simulink model "VFOC"  (R2015a)
settings: Solver=ode45  StartTime=0.0  StopTime=10.0  RelTol=1e-3
values from neighbouring files (symbols this model uses):
  C = 2350e-6    (= 0.00235)    [VOC_param.m]    (also in VOC_param_paper.m = 0.0022; controller_parameters.m = 0.0022; power_control_param.m = 0.02)
  Hp = 0    [VOC_param.m]    (also in power_control_param.m = 20)
  Hq = 0    [VOC_param.m]    (also in power_control_param.m)
  I = 0.1    [power_control_param.m]
  Ka = fluxeff    (= 0.15)    [VOC_param.m]    (also in VOC_param_paper.m; power_control_param.m)
  L = 8e-3    (= 0.008)    [VOC_param.m]    (also in VOC_param_paper.m = 0.003; controller_parameters.m = 0.003; current_controller_param.m = 0.005; power_control_param.m = 0.1)
  p = 4    [VOC_param.m]    (also in VOC_param_paper.m; power_control_param.m)
  P = 1    [power_control_param.m]
  R = 0.1    [VOC_param.m]    (also in VOC_param_paper.m = 0.05; controller_parameters.m = 0.05; current_controller_param.m; power_control_param.m = 0)
  RL = 120    [VOC_param.m]    (also in VOC_param_paper.m = 150; power_control_param.m = 80)
  rpm2radps = pi/30    (= 0.10471975512)    [VOC_param.m]    (also in VOC_param_paper.m; power_control_param.m)
  U = 311    [VOC_param.m]    (also in power_control_param.m)
  Udcref = 120    [VOC_param.m]    (also in VOC_param_paper.m; power_control_param.m = 10)
  w = 2*pi*f    (= 314.159265359)    [VOC_param.m]    (also in controller_parameters.m; current_controller_param.m; power_control_param.m)
libraries: simulink x2
settings Model: Creator=rblan  LastModifiedBy=rblan

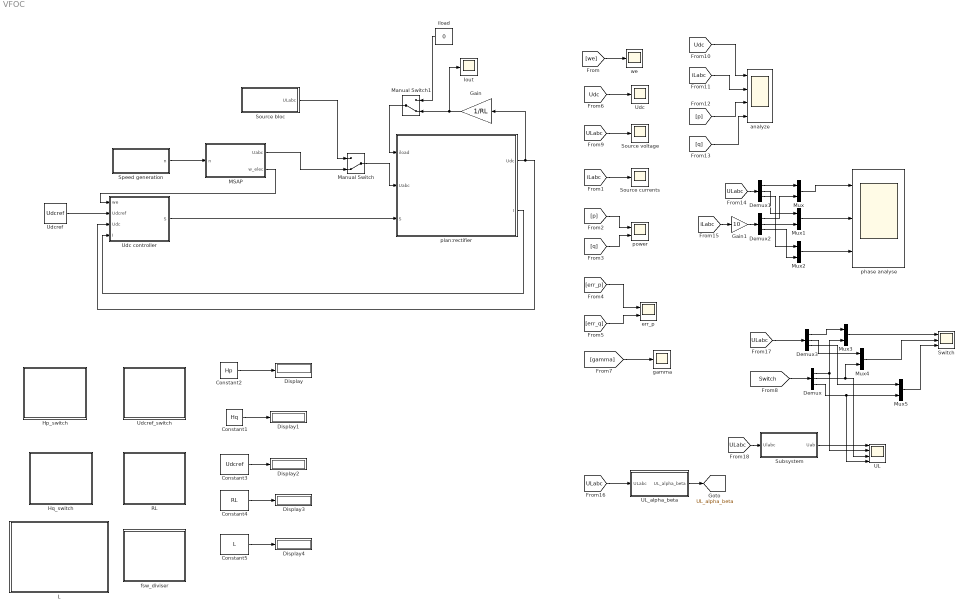
== system VFOC ==
  Constant1 : Constant  Value=Hq
  Constant2 : Constant  Value=Hp
  Constant3 : Constant  Value=Udcref
  Constant4 : Constant  Value=RL
  Constant5 : Constant  Value=L
  Demux{,1..3} (4 alike) : Demux  Outputs=3
  Display{,1..4} (5 alike) : Display
  Gain : Gain  Gain=1/RL
  Gain1 : Gain  Gain=10
  Hp_switch : Subsystem  DialogController=hmiCreateDDGDialog  IsWebBlock=on  mask(MathWorksWebBlock){webBlockId=fe3dbe73-a954-44d9-9dcb-6f2e0f6423d3, webBlockType=continuousknob, ShowInLibBrowser=on, ShowInitialText=on, HMISrcModelName=VFOC}
      mask prompts: webBlockId "WebBlock Id"; webBlockType "WebBlock Type"; HMISrcModelName "Source Model"
      mask Help: helpview([docroot '/mapfiles/simulink.map'], 'hmi_knob')
      mask Display:
      | if strcmp(get_param(bdroot(gcb),'BlockDiagramType'), 'library')
      |     image([(matlabroot) '/toolbox/simulink/hmi/icons/ContinuousKnob.png']);
      | end
  Hq_switch : Subsystem  DialogController=hmiCreateDDGDialog  IsWebBlock=on  mask(MathWorksWebBlock){webBlockId=a89797ed-0246-4893-8a6d-d9668782cbd3, webBlockType=continuousknob, ShowInLibBrowser=on, ShowInitialText=on, HMISrcModelName=VFOC}
      mask prompts: webBlockId "WebBlock Id"; webBlockType "WebBlock Type"; HMISrcModelName "Source Model"
      mask Help: helpview([docroot '/mapfiles/simulink.map'], 'hmi_knob')
      mask Display:
      | if strcmp(get_param(bdroot(gcb),'BlockDiagramType'), 'library')
      |     image([(matlabroot) '/toolbox/simulink/hmi/icons/ContinuousKnob.png']);
      | end
  Iout : Scope
      settings: YMin=0.2275  YMax=0.2575  SaveName=ScopeData13
  L : Subsystem  DialogController=hmiCreateDDGDialog  IsWebBlock=on  mask(MathWorksWebBlock){webBlockId=ffd7f022-e8a1-4d04-9927-9b962ba217d4, webBlockType=continuousknob, ShowInLibBrowser=on, ShowInitialText=on, HMISrcModelName=VFOC}
      mask prompts: webBlockId "WebBlock Id"; webBlockType "WebBlock Type"; HMISrcModelName "Source Model"
      mask Help: helpview([docroot '/mapfiles/simulink.map'], 'hmi_knob')
      mask Display:
      | if strcmp(get_param(bdroot(gcb),'BlockDiagramType'), 'library')
      |     image([(matlabroot) '/toolbox/simulink/hmi/icons/ContinuousKnob.png']);
      | end
  MSAP : Subsystem
  Manual Switch : ManualSwitch  CurrentSetting=0
  Manual Switch1 : ManualSwitch  CurrentSetting=0
  Mux{,1..5} (6 alike) : Mux  Inputs=2
  RL : Subsystem  DialogController=hmiCreateDDGDialog  IsWebBlock=on  mask(MathWorksWebBlock){webBlockId=6d3a3d3f-09f6-4f12-a865-f4fdcd28252a, webBlockType=continuousknob, ShowInLibBrowser=on, ShowInitialText=on, HMISrcModelName=VFOC}
      mask prompts: webBlockId "WebBlock Id"; webBlockType "WebBlock Type"; HMISrcModelName "Source Model"
      mask Help: helpview([docroot '/mapfiles/simulink.map'], 'hmi_knob')
      mask Display:
      | if strcmp(get_param(bdroot(gcb),'BlockDiagramType'), 'library')
      |     image([(matlabroot) '/toolbox/simulink/hmi/icons/ContinuousKnob.png']);
      | end
  Source bloc : Subsystem
  Source currents : Scope
      settings: TimeRange=2  YMin=-3  YMax=2.25  SaveName=Iabc
  "Source voltage " : Scope
      settings: TimeRange=0.06239913932221623  YMin=-20  YMax=20  SaveName=Uabc
  Speed generation : Subsystem
  Subsystem : Subsystem
  Switch : Scope  NumInputPorts=3
      settings: YMin=-2~-5~-5  YMax=5~5~5  SaveName=ScopeData8
  "UL " : Scope  NumInputPorts=4
      settings: YMin=-2~-5~-5~-5  YMax=5~5~5~5  SaveName=ScopeData19
  UL_alpha_beta : Subsystem
  Udc : Scope
      settings: TimeRange=3  YMin=15  YMax=21.5  SaveName=Udc
  Udc controller : Subsystem
  Udcref : Constant  Value=Udcref
  Udcref_switch : Subsystem  DialogController=hmiCreateDDGDialog  IsWebBlock=on  mask(MathWorksWebBlock){webBlockId=8174ab9b-ad42-417a-b04d-5b98e4451fc4, webBlockType=continuousknob, ShowInLibBrowser=on, ShowInitialText=on, HMISrcModelName=VFOC}
      mask prompts: webBlockId "WebBlock Id"; webBlockType "WebBlock Type"; HMISrcModelName "Source Model"
      mask Help: helpview([docroot '/mapfiles/simulink.map'], 'hmi_knob')
      mask Display:
      | if strcmp(get_param(bdroot(gcb),'BlockDiagramType'), 'library')
      |     image([(matlabroot) '/toolbox/simulink/hmi/icons/ContinuousKnob.png']);
      | end
  analyze : Scope  NumInputPorts=4
      settings: TimeRange=0.06239913932221623  YMin=0~-1.75~-25~-5  YMax=20~1.75~100~100  SaveName=Uabc1
  err_p : Scope  NumInputPorts=2
      settings: TimeRange=2  YMin=-40~-65  YMax=40~0  SaveName=err_p
  fsw_diviser : Subsystem  DialogController=hmiCreateDDGDialog  IsWebBlock=on  mask(MathWorksWebBlock){webBlockId=92bd8738-3137-464c-9b2e-3fda7a42618d, webBlockType=continuousknob, ShowInLibBrowser=on, ShowInitialText=on, HMISrcModelName=VFOC}
      mask prompts: webBlockId "WebBlock Id"; webBlockType "WebBlock Type"; HMISrcModelName "Source Model"
      mask Help: helpview([docroot '/mapfiles/simulink.map'], 'hmi_knob')
      mask Display:
      | if strcmp(get_param(bdroot(gcb),'BlockDiagramType'), 'library')
      |     image([(matlabroot) '/toolbox/simulink/hmi/icons/ContinuousKnob.png']);
      | end
  gamma : Scope
      settings: YMin=-2  SaveName=ScopeData5
  iload : Constant  Value=0
  phase analyse : Scope  NumInputPorts=3
      settings: TimeRange=0.06239913932221623  YMin=-30~-30~-30  YMax=30~30~30  SaveName=Uabc2
  plan:rectifier : Subsystem
  "power " : Scope  NumInputPorts=2
      settings: YMin=-20~-5  YMax=75~47.5  SaveName=p
  we : Scope
      settings: YMin=119.381  YMax=131.947  SaveName=ScopeData10
  tag scope: UL_alpha_beta=global
  wires:
  [iLabc] -> Source currents/1
  [p] -> "power "/1
  [q] -> "power "/2
  [err_p] -> err_p/1
  [Udc] -> Udc/1
  [gamma] -> gamma/1
  Manual Switch/1 -> plan:rectifier/2(Uabc)
  [ULabc] -> "Source voltage "/1
  Source bloc/1(ULabc) -> Manual Switch/1
  [we] -> we/1
  Udcref/1 -> Udc controller/2(Udcref)
  plan:rectifier/1(Udc) -> Gain/1, Udc controller/3(Udc)
  MSAP/1(Uabc) -> Manual Switch/2
  Speed generation/1(n) -> MSAP/1(n)
  MSAP/2(w_elec) -> Udc controller/1(we)
  [Switch] -> Demux/1
  plan:rectifier/2(I) -> Udc controller/4(I)
  Udc controller/1(S) -> plan:rectifier/3(S)
  iload/1 -> Manual Switch1/1
  Gain/1 -> Iout/1, Manual Switch1/2
  Manual Switch1/1 -> plan:rectifier/1(iload)
  [Udc] -> analyze/1
  [iLabc] -> analyze/2
  [p] -> analyze/3
  [q] -> analyze/4
  [ULabc] -> Demux1/1
  [iLabc] -> Gain1/1
  Mux/1 -> phase analyse/1
  Demux1/1 -> Mux/1
  Demux2/1 -> Mux/2
  Mux1/1 -> phase analyse/2
  Mux2/1 -> phase analyse/3
  Demux1/2 -> Mux1/1
  Demux2/2 -> Mux1/2
  Demux1/3 -> Mux2/1
  Demux2/3 -> Mux2/2
  Gain1/1 -> Demux2/1
  [err_q] -> err_p/2
  Constant2/1 -> Display/1
  Constant1/1 -> Display1/1
  Constant3/1 -> Display2/1
  Constant4/1 -> Display3/1
  Constant5/1 -> Display4/1
  [ULabc] -> UL_alpha_beta/1(ULabc)
  UL_alpha_beta/1(UL_alpha_beta) -> [UL_alpha_beta]
  [ULabc] -> Demux3/1
  Mux3/1 -> Switch/1
  Demux3/1 -> Mux3/1
  Demux/1 -> Mux3/2, "UL "/2
  Mux4/1 -> Switch/2
  Demux3/2 -> Mux4/1
  Demux/2 -> "UL "/3, Mux4/2
  Mux5/1 -> Switch/3
  Demux3/3 -> Mux5/1
  Demux/3 -> "UL "/4, Mux5/2
  [ULabc] -> Subsystem/1(Ulabc)
  Subsystem/1("Uab ") -> "UL "/1

== system VFOC/Hp_switch ==

== system VFOC/Hq_switch ==

== system VFOC/L ==

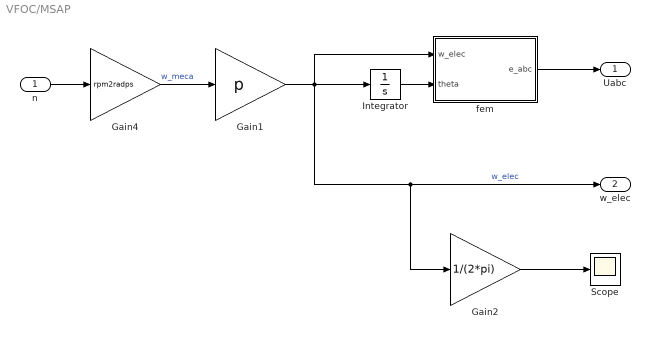
== system VFOC/MSAP ==
  n : Inport
  Gain1 : Gain  Gain=p
  Gain2 : Gain  Gain=1/(2*pi)
  Gain4 : Gain  Gain=rpm2radps
  Integrator : Integrator
  Scope : Scope
      settings: YMin=19  YMax=21  SaveName=ScopeData9
  fem : Subsystem
  Uabc : Outport
  w_elec : Outport  Port=2
  wires:
  Integrator/1 -> fem/2(theta)
  Gain1/1 -> Integrator/1, Gain2/1, w_elec/1, fem/1(w_elec)  "w_elec"
  n/1 -> Gain4/1
  Gain4/1 -> Gain1/1  "w_meca"
  fem/1(e_abc) -> Uabc/1
  Gain2/1 -> Scope/1

== system VFOC/RL ==

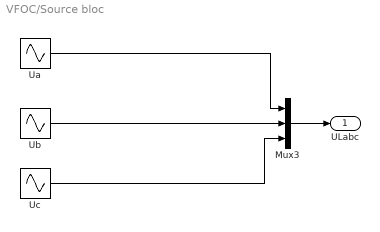
== system VFOC/Source bloc ==
  Mux3 : Mux  Inputs=3
  Ua : Sin  Amplitude=U  Frequency=w  SampleTime=0
  Ub : Sin  Amplitude=U  Frequency=w  Phase=-2*pi/3  SampleTime=0
  Uc : Sin  Amplitude=U  Frequency=w  Phase=-4*pi/3  SampleTime=0
  ULabc : Outport
  wires:
  Ua/1 -> Mux3/1
  Uc/1 -> Mux3/3
  Ub/1 -> Mux3/2
  Mux3/1 -> ULabc/1

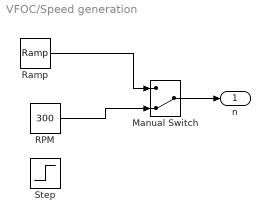
== system VFOC/Speed generation ==
  Manual Switch : ManualSwitch  CurrentSetting=0
  RPM : Constant  Value=300
  Ramp : simulink/Sources/Ramp  slope=50  start=0  X0=100
  Step : Step  Time=1.5  After=0  SampleTime=0
  n : Outport
  wires:
  Ramp/1 -> Manual Switch/1
  Manual Switch/1 -> n/1
  RPM/1 -> Manual Switch/2

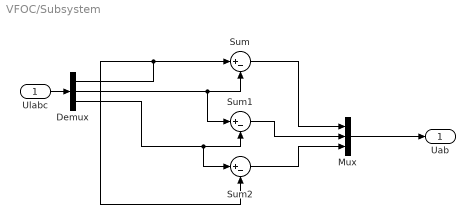
== system VFOC/Subsystem ==
  Ulabc : Inport
  Demux : Demux  Outputs=3
  Mux : Mux  Inputs=3
  Sum : Sum  Inputs=|+-
  Sum1 : Sum  Inputs=|+-
  Sum2 : Sum  Inputs=|+-
  "Uab " : Outport
  wires:
  Ulabc/1 -> Demux/1
  Demux/1 -> Sum/1, Sum2/2
  Demux/2 -> Sum1/1, Sum/2
  Demux/3 -> Sum2/1, Sum1/2
  Mux/1 -> "Uab "/1
  Sum/1 -> Mux/1
  Sum1/1 -> Mux/2
  Sum2/1 -> Mux/3

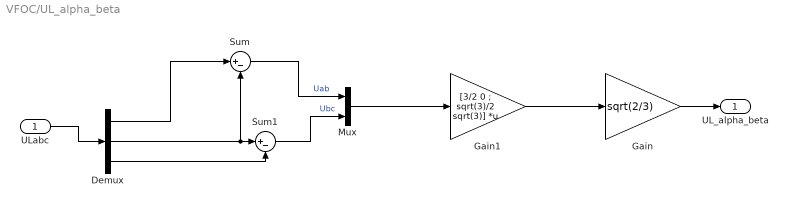
== system VFOC/UL_alpha_beta ==
  ULabc : Inport
  Demux : Demux  Outputs=3
  Gain : Gain  Gain=sqrt(2/3)
  Gain1 : Gain  Gain=[3/2 0 ; sqrt(3)/2 sqrt(3)]  Multiplication=Matrix(K*u)
  Mux : Mux  Inputs=2
  Sum : Sum  Inputs=|+-
  Sum1 : Sum  Inputs=|+-
  UL_alpha_beta : Outport
  wires:
  ULabc/1 -> Demux/1
  Demux/1 -> Sum/1
  Demux/2 -> Sum/2, Sum1/1
  Demux/3 -> Sum1/2
  Gain/1 -> UL_alpha_beta/1
  Gain1/1 -> Gain/1
  Sum/1 -> Mux/1  "Uab"
  Sum1/1 -> Mux/2  "Ubc"
  Mux/1 -> Gain1/1

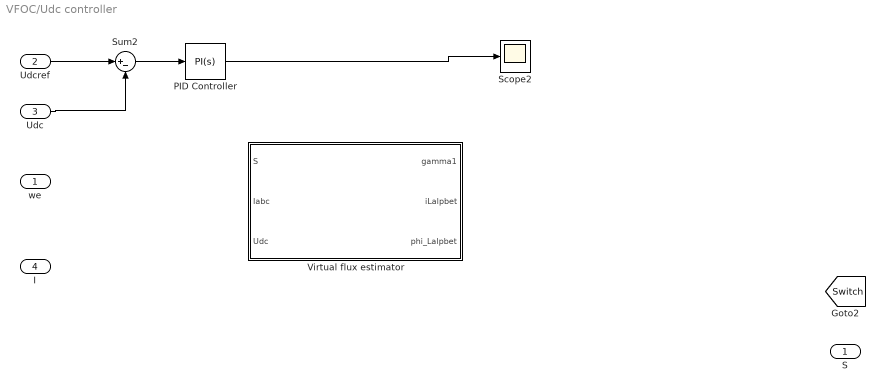
== system VFOC/Udc controller ==
  we : Inport
  Udcref : Inport  Port=2
  Udc : Inport  Port=3
  I : Inport  Port=4
  PID Controller : simulink/Continuous/PID Controller  Controller=PI  TimeDomain=Continuous-time  SampleTime=-1  IntegratorMethod=Forward Euler  FilterMethod=Forward Euler  Form=Parallel  UseFilter=on  ControllerParametersSource=internal  P=P  I=I  D=0  N=100  InitialConditionSource=internal  InitialConditionForIntegrator=0  InitialConditionForFilter=0  ExternalReset=none  LimitOutput=off  UpperSaturationLimit=inf  LowerSaturationLimit=-inf  LinearizeAsGain=on  AntiWindupMode=none  Kb=1  TrackingMode=off  Kt=1  PParamMin=[]  PParamMax=[]  IParamMin=[]  IParamMax=[]  DParamMin=[]  DParamMax=[]  NParamMin=[]  NParamMax=[]  KbParamMin=[]  KbParamMax=[]  KtParamMin=[]  KtParamMax=[]  POutMin=[]  POutMax=[]  IOutMin=[]  IOutMax=[]  DOutMin=[]  DOutMax=[]  NOutMin=[]  NOutMax=[]  KbOutMin=[]  KbOutMax=[]  KtOutMin=[]  KtOutMax=[]  IntegratorOutMin=[]  IntegratorOutMax=[]  FilterOutMin=[]  FilterOutMax=[]  SumOutMin=[]  SumOutMax=[]  SumI1OutMin=[]  SumI1OutMax=[]  SumI2OutMin=[]  SumI2OutMax=[]  SumI3OutMin=[]  SumI3OutMax=[]  SumDOutMin=[]  SumDOutMax=[]  SaturationOutMin=[]  SaturationOutMax=[]  IntegratorContinuousStateAttributes=''  IntegratorStateMustResolveToSignalObject=off  IntegratorRTWStateStorageClass=Auto  FilterContinuousStateAttributes=''  FilterStateMustResolveToSignalObject=off  FilterRTWStateStorageClass=Auto  DifferentiatorICPrevScaledInput=0  DifferentiatorOutMin=[]  DifferentiatorOutMax=[]
  Scope2 : Scope
      settings: YMin=230  YMax=265  SaveName=ScopeData17
  Sum2 : Sum  Inputs=|+-
  Virtual flux estimator : Subsystem
  S : Outport
  tag scope: Switch=global
  wires:
  ? -> S/1, [Switch]
  Udc/1 -> Sum2/2
  Sum2/1 -> PID Controller/1
  Udcref/1 -> Sum2/1
  PID Controller/1 -> Scope2/1

== system VFOC/Udcref_switch ==

== system VFOC/fsw_diviser ==

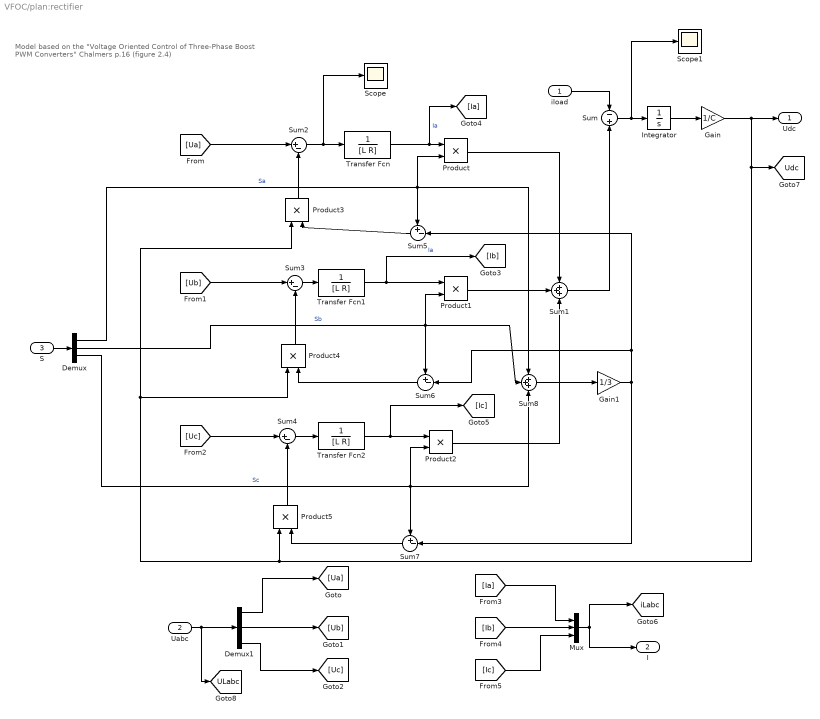
== system VFOC/plan:rectifier ==
  note: Model based on the "Voltage Oriented Control of Three‐Phase
      | Boost PWM Converters" Chalmers p.16 (figure 2.4)
  iload : Inport
  Uabc : Inport  Port=2
  S : Inport  Port=3
  Demux : Demux  Outputs=3
  Demux1 : Demux  Outputs=3
  Gain : Gain  Gain=1/C
  Gain1 : Gain  Gain=1/3
  Integrator : Integrator
  Mux : Mux  Inputs=3
  Product{,1..5} (6 alike) : Product
  Scope : Scope
      settings: SaveName=ScopeData14
  Scope1 : Scope
      settings: SaveName=ScopeData12
  Sum : Sum  Inputs=-|+
  Sum1 : Sum  Inputs=+++
  Sum2 : Sum  Inputs=|+-
  Sum3 : Sum  Inputs=|+-
  Sum4 : Sum  Inputs=|+-
  Sum5 : Sum  Inputs=+-|
  Sum6 : Sum  Inputs=+-|
  Sum7 : Sum  Inputs=+-|
  Sum8 : Sum  Inputs=+++
  Transfer Fcn : TransferFcn  Denominator=[L R]  ContinuousStateAttributes='Ia'
  Transfer Fcn1 : TransferFcn  Denominator=[L R]
  Transfer Fcn2 : TransferFcn  Denominator=[L R]
  Udc : Outport
  I : Outport  Port=2
  tag scope: ULabc=global, Udc=global, iLabc=global
  wires:
  Gain/1 -> [Udc], Product5/1, Product3/1, Product4/1, Udc/1
  Integrator/1 -> Gain/1
  iload/1 -> Sum/1
  Sum1/1 -> Sum/2
  Product/1 -> Sum1/1
  Product1/1 -> Sum1/2
  Product2/1 -> Sum1/3
  Transfer Fcn/1 -> [Ia], Product/1  "Ia"
  Transfer Fcn1/1 -> [Ib], Product1/1  "Ia"
  Transfer Fcn2/1 -> [Ic], Product2/1
  Sum2/1 -> Scope/1, Transfer Fcn/1
  [Ua] -> Sum2/1
  Product3/1 -> Sum2/2
  Sum3/1 -> Transfer Fcn1/1
  Sum4/1 -> Transfer Fcn2/1
  [Ub] -> Sum3/1
  [Uc] -> Sum4/1
  Demux/1 -> Sum8/1, Product/2, Sum5/1  "Sa"
  Demux/2 -> Sum6/1, Sum8/2, Product1/2  "Sb"
  Demux/3 -> Sum8/3, Sum7/1, Product2/2  "Sc"
  Product4/1 -> Sum3/2
  Product5/1 -> Sum4/2
  Sum5/1 -> Product3/2
  Sum6/1 -> Product4/2
  Sum7/1 -> Product5/2
  Sum/1 -> Scope1/1, Integrator/1
  Sum8/1 -> Gain1/1
  Gain1/1 -> Sum6/2, Sum5/2, Sum7/2
  S/1 -> Demux/1
  Uabc/1 -> [ULabc], Demux1/1
  Demux1/1 -> [Ua]
  Demux1/2 -> [Ub]
  Demux1/3 -> [Uc]
  Mux/1 -> [iLabc], I/1
  [Ia] -> Mux/1
  [Ib] -> Mux/2
  [Ic] -> Mux/3

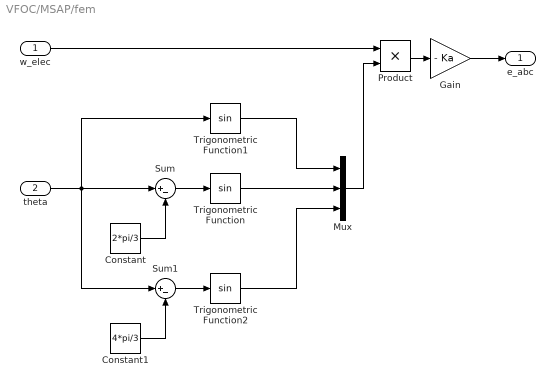
== system VFOC/MSAP/fem ==
  w_elec : Inport
  theta : Inport  Port=2
  Constant : Constant  Value=2*pi/3
  Constant1 : Constant  Value=4*pi/3
  Gain : Gain  Gain=- Ka
  Mux : Mux  Inputs=3
  Product : Product
  Sum : Sum  Inputs=|+-
  Sum1 : Sum  Inputs=|+-
  Trigonometric Function : Trigonometry
  Trigonometric Function1 : Trigonometry
  Trigonometric Function2 : Trigonometry
  e_abc : Outport
  wires:
  Mux/1 -> Product/2
  theta/1 -> Sum/1, Trigonometric Function1/1, Sum1/1
  Constant1/1 -> Sum1/2
  Sum1/1 -> Trigonometric Function2/1
  Constant/1 -> Sum/2
  Sum/1 -> Trigonometric Function/1
  w_elec/1 -> Product/1
  Product/1 -> Gain/1
  Gain/1 -> e_abc/1
  Trigonometric Function1/1 -> Mux/1
  Trigonometric Function2/1 -> Mux/3
  Trigonometric Function/1 -> Mux/2

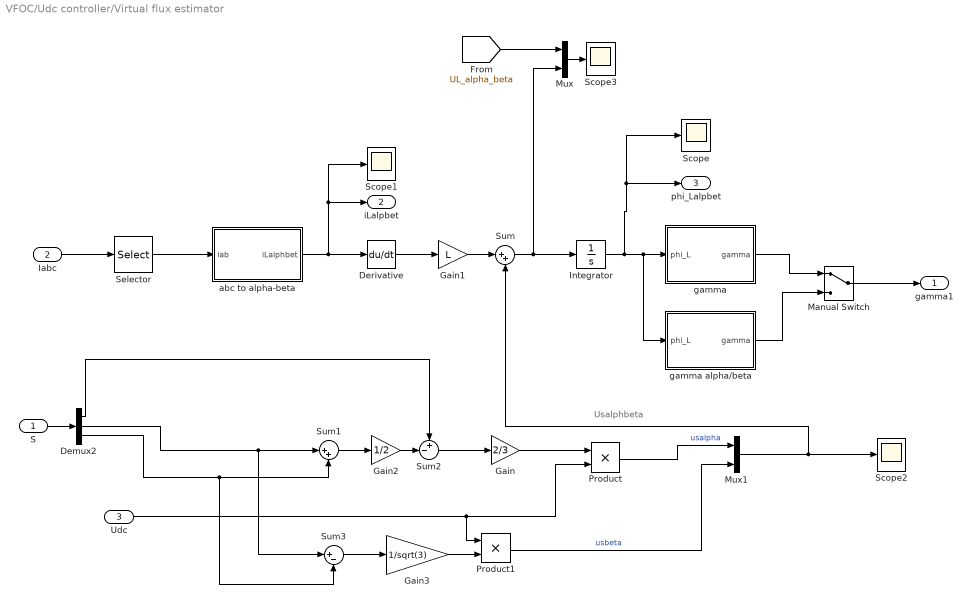
== system VFOC/Udc controller/Virtual flux estimator ==
  note: Usalphbeta
  S : Inport
  Iabc : Inport  Port=2
  Udc : Inport  Port=3
  Demux2 : Demux  Outputs=3
  Derivative : Derivative
  Gain : Gain  Gain=2/3
  Gain1 : Gain  Gain=L
  Gain2 : Gain  Gain=1/2
  Gain3 : Gain  Gain=1/sqrt(3)
  Integrator : Integrator
  Manual Switch : ManualSwitch
  Mux : Mux  Inputs=2
  Mux1 : Mux  Inputs=2
  Product : Product
  Product1 : Product
  Scope{,1..3} (4 alike) : Scope
      Scope settings: ShowLegends=on  YMin=-0.45  YMax=0.45
      Scope1 settings: YMin=-450  YMax=450
      Scope2 settings: ShowLegends=on  YMin=-8  YMax=8  SaveName=ScopeData4
      Scope3 settings: ShowLegends=on  YMin=-40  YMax=40  SaveName=ScopeData11
  Selector : Selector  InputPortWidth=3  Indices=[1 2]
  Sum : Sum  Inputs=|++
  Sum1 : Sum  Inputs=|++
  Sum2 : Sum  Inputs=+-|
  Sum3 : Sum  Inputs=|+-
  abc to alpha-beta : Subsystem
  gamma : Subsystem
  gamma alpha/beta : Subsystem
  gamma1 : Outport
  iLalpbet : Outport  Port=2
  phi_Lalpbet : Outport  Port=3
  wires:
  abc to alpha-beta/1(iLalphbet) -> Derivative/1, Scope1/1, iLalpbet/1
  Gain1/1 -> Sum/1
  Demux2/2 -> Sum3/1, Sum1/1
  Demux2/3 -> Sum3/2, Sum1/2
  Sum1/1 -> Gain2/1
  Gain2/1 -> Sum2/2
  Demux2/1 -> Sum2/1
  Sum2/1 -> Gain/1
  Gain/1 -> Product/1
  Udc/1 -> Product/2, Product1/1
  Product/1 -> Mux1/1  "usalpha"
  Sum3/1 -> Gain3/1
  Gain3/1 -> Product1/2
  Product1/1 -> Mux1/2  "usbeta"
  Integrator/1 -> gamma alpha/beta/1(phi_L), gamma/1(phi_L), Scope/1, phi_Lalpbet/1
  Mux1/1 -> Scope2/1, Sum/2
  S/1 -> Demux2/1
  Selector/1 -> abc to alpha-beta/1(iab)
  Iabc/1 -> Selector/1
  Sum/1 -> Mux/2, Integrator/1
  Derivative/1 -> Gain1/1
  gamma/1(gamma) -> Manual Switch/1
  gamma alpha/beta/1(gamma) -> Manual Switch/2
  Manual Switch/1 -> gamma1/1
  Mux/1 -> Scope3/1
  [UL_alpha_beta] -> Mux/1

== system VFOC/Udc controller/Virtual flux estimator/abc to alpha-beta ==
  iab : Inport
  Gain : Gain  Gain=sqrt(2/3)
  Gain1 : Gain  Gain=[3/2 0 ; sqrt(3)/2 sqrt(3)]  Multiplication=Matrix(K*u)
  iLalphbet : Outport
  wires:
  Gain1/1 -> Gain/1
  iab/1 -> Gain1/1
  Gain/1 -> iLalphbet/1

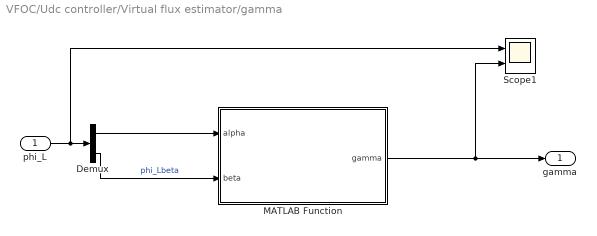
== system VFOC/Udc controller/Virtual flux estimator/gamma ==
  phi_L : Inport
  Demux : Demux  Outputs=2
  MATLAB Function : MATLAB Function  TreatAsAtomicUnit=on
  Scope1 : Scope  NumInputPorts=2
      settings: ShowLegends=on  YMin=-0.3~0  YMax=0.3~6.5  SaveName=ScopeData3
  gamma : Outport
  wires:
  phi_L/1 -> Scope1/1, Demux/1
  Demux/1 -> MATLAB Function/1(alpha)
  Demux/2 -> MATLAB Function/2(beta)  "phi_Lbeta"
  MATLAB Function/1(gamma) -> Scope1/2, gamma/1

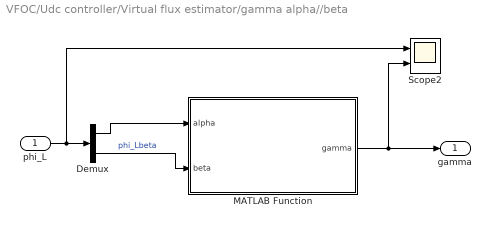
== system VFOC/Udc controller/Virtual flux estimator/gamma alpha//beta ==
  phi_L : Inport
  Demux : Demux  Outputs=2
  MATLAB Function : MATLAB Function  TreatAsAtomicUnit=on
  Scope2 : Scope  NumInputPorts=2
      settings: YMin=-1.75~-500  YMax=1.75~300  SaveName=ScopeData15
  gamma : Outport
  wires:
  phi_L/1 -> Scope2/1, Demux/1
  Demux/1 -> MATLAB Function/1(alpha)
  Demux/2 -> MATLAB Function/2(beta)  "phi_Lbeta"
  MATLAB Function/1(gamma) -> gamma/1, Scope2/2

== matlab function VFOC/Udc controller/Virtual flux estimator/gamma/MATLAB Function ==
  data: alpha input; gamma output; beta input
function gamma = gamma_estimator(alpha,beta)
%#codegen

gamma = 0 ; 
gamma = atan(beta/alpha)+pi/2 ; 

if (alpha<0 )
    gamma = gamma +pi ; 
end 

if (beta<0 && alpha> 0 ) 
    gamma = gamma +2*pi ; 
end 

if (gamma>(2*pi) )
    gamma = gamma -2*pi ; 
end

== matlab function VFOC/Udc controller/Virtual flux estimator/gamma alpha//beta/MATLAB Function ==
  data: alpha input; gamma output; beta input
function gamma = gamma_estimator(alpha,beta)
%#codegen

gamma = 0 ; 
gamma = atan(beta/alpha) ; 

if (alpha<0 )
    gamma = gamma +pi ; 
end 

if (beta<0 && alpha> 0 ) 
    gamma = gamma +2*pi ; 
end
